simulink model "IEEE14_bus_system_2"  (R2024a)
settings: Solver=VariableStepAuto  StartTime=0.0  StopTime=0.2  RelTol=1e-3
libraries: spsThreePhaseSeriesRLCBranchLib x120, spsThreePhaseVIMeasurementLib x51, spsGroundLib x40, spsLoadFlowBusLib x33, spsThreePhaseSeriesRLCLoadLib x24, spsThreePhaseSourceLib x10, spsThreePhaseTransformerTwoWindingsLib x5, spspowerguiLib x2
(part 3 of 3)

== system IEEE14_bus_system_2/Line 4-3 ==
  B1 : spsThreePhaseSeriesRLCBranchLib/Three-Phase Series RLC Branch  LConnTagsString=A|B|C  RConnTagsString=A|B|C  BranchType=C  Resistance=1e-6  Inductance=1e-3  Capacitance=B/(2*pi*F)  Measurements=None
  B2 : spsThreePhaseSeriesRLCBranchLib/Three-Phase Series RLC Branch  LConnTagsString=A|B|C  RConnTagsString=A|B|C  BranchType=C  Resistance=1e-6  Inductance=1e-3  Capacitance=B/(2*pi*F)  Measurements=None
  Ground : spsGroundLib/Ground  LConnTagsString=a
  RL : spsThreePhaseSeriesRLCBranchLib/Three-Phase Series RLC Branch  LConnTagsString=A|B|C  RConnTagsString=A|B|C  BranchType=RL  Resistance=R  Inductance=xL/(2*pi*F)  Capacitance=1e-6  Measurements=None
  A : PMIOPort  Side=Left
  B : PMIOPort  Port=2  Side=Left
  C : PMIOPort  Port=3  Side=Left
  a : PMIOPort  Port=4  Side=Right
  b : PMIOPort  Port=5  Side=Right
  c : PMIOPort  Port=6  Side=Right
  connections:
  RL/LConn1 -- A/RConn1 -- B1/LConn1
  RL/RConn1 -- a/RConn1 -- B2/LConn1
  RL/LConn2 -- B/RConn1 -- B1/LConn2
  RL/RConn2 -- b/RConn1 -- B2/LConn2
  RL/RConn3 -- B2/LConn3 -- c/RConn1
  RL/LConn3 -- B1/LConn3 -- C/RConn1
  B1/RConn1 -- B1/RConn2 -- B1/RConn3 -- B2/RConn1 -- B2/RConn2 -- B2/RConn3 -- Ground/LConn1

== system IEEE14_bus_system_2/Line 4-5 ==
  B1 : spsThreePhaseSeriesRLCBranchLib/Three-Phase Series RLC Branch  LConnTagsString=A|B|C  RConnTagsString=A|B|C  BranchType=C  Resistance=0  Inductance=1e-3  Capacitance=B/(2*pi*F)  Measurements=None
  B2 : spsThreePhaseSeriesRLCBranchLib/Three-Phase Series RLC Branch  LConnTagsString=A|B|C  RConnTagsString=A|B|C  BranchType=C  Resistance=1e-6  Inductance=1e-3  Capacitance=B/(2*pi*F)  Measurements=None
  Ground : spsGroundLib/Ground  LConnTagsString=a
  RL : spsThreePhaseSeriesRLCBranchLib/Three-Phase Series RLC Branch  LConnTagsString=A|B|C  RConnTagsString=A|B|C  BranchType=RL  Resistance=R  Inductance=xL/(2*pi*F)  Capacitance=1e-6  Measurements=None
  A : PMIOPort  Side=Left
  B : PMIOPort  Port=2  Side=Left
  C : PMIOPort  Port=3  Side=Left
  a : PMIOPort  Port=4  Side=Right
  b : PMIOPort  Port=5  Side=Right
  c : PMIOPort  Port=6  Side=Right
  connections:
  RL/LConn1 -- A/RConn1 -- B1/LConn1
  RL/RConn1 -- a/RConn1 -- B2/LConn1
  RL/LConn2 -- B/RConn1 -- B1/LConn2
  RL/RConn2 -- b/RConn1 -- B2/LConn2
  RL/RConn3 -- B2/LConn3 -- c/RConn1
  RL/LConn3 -- B1/LConn3 -- C/RConn1
  B1/RConn1 -- B1/RConn2 -- B1/RConn3 -- B2/RConn1 -- B2/RConn2 -- B2/RConn3 -- Ground/LConn1

== system IEEE14_bus_system_2/Line 4-7 ==
  B1 : spsThreePhaseSeriesRLCBranchLib/Three-Phase Series RLC Branch  LConnTagsString=A|B|C  RConnTagsString=A|B|C  BranchType=C  Resistance=1e-6  Inductance=1e-3  Capacitance=B/(2*pi*F)  Measurements=None
  B2 : spsThreePhaseSeriesRLCBranchLib/Three-Phase Series RLC Branch  LConnTagsString=A|B|C  RConnTagsString=A|B|C  BranchType=C  Resistance=1e-6  Inductance=1e-3  Capacitance=B/(2*pi*F)  Measurements=None
  Ground : spsGroundLib/Ground  LConnTagsString=a
  RL : spsThreePhaseSeriesRLCBranchLib/Three-Phase Series RLC Branch  LConnTagsString=A|B|C  RConnTagsString=A|B|C  BranchType=RL  Resistance=R  Inductance=xL/(2*pi*F)  Capacitance=1e-6  Measurements=None
  A : PMIOPort  Side=Left
  B : PMIOPort  Port=2  Side=Left
  C : PMIOPort  Port=3  Side=Left
  a : PMIOPort  Port=4  Side=Right
  b : PMIOPort  Port=5  Side=Right
  c : PMIOPort  Port=6  Side=Right
  connections:
  RL/LConn1 -- A/RConn1 -- B1/LConn1
  RL/RConn1 -- a/RConn1 -- B2/LConn1
  RL/LConn2 -- B/RConn1 -- B1/LConn2
  RL/RConn2 -- b/RConn1 -- B2/LConn2
  RL/RConn3 -- B2/LConn3 -- c/RConn1
  RL/LConn3 -- B1/LConn3 -- C/RConn1
  B1/RConn1 -- B1/RConn2 -- B1/RConn3 -- B2/RConn1 -- B2/RConn2 -- B2/RConn3 -- Ground/LConn1

== system IEEE14_bus_system_2/Line 4-9 ==
  B1 : spsThreePhaseSeriesRLCBranchLib/Three-Phase Series RLC Branch  LConnTagsString=A|B|C  RConnTagsString=A|B|C  BranchType=C  Resistance=1e-6  Inductance=1e-3  Capacitance=B/(2*pi*F)  Measurements=None
  B2 : spsThreePhaseSeriesRLCBranchLib/Three-Phase Series RLC Branch  LConnTagsString=A|B|C  RConnTagsString=A|B|C  BranchType=C  Resistance=1e-6  Inductance=1e-3  Capacitance=B/(2*pi*F)  Measurements=None
  Ground : spsGroundLib/Ground  LConnTagsString=a
  RL : spsThreePhaseSeriesRLCBranchLib/Three-Phase Series RLC Branch  LConnTagsString=A|B|C  RConnTagsString=A|B|C  BranchType=RL  Resistance=R  Inductance=xL/(2*pi*F)  Capacitance=1e-6  Measurements=None
  A : PMIOPort  Side=Left
  B : PMIOPort  Port=2  Side=Left
  C : PMIOPort  Port=3  Side=Left
  a : PMIOPort  Port=4  Side=Right
  b : PMIOPort  Port=5  Side=Right
  c : PMIOPort  Port=6  Side=Right
  connections:
  RL/LConn1 -- A/RConn1 -- B1/LConn1
  RL/RConn1 -- a/RConn1 -- B2/LConn1
  RL/LConn2 -- B/RConn1 -- B1/LConn2
  RL/RConn2 -- b/RConn1 -- B2/LConn2
  RL/RConn3 -- B2/LConn3 -- c/RConn1
  RL/LConn3 -- B1/LConn3 -- C/RConn1
  B1/RConn1 -- B1/RConn2 -- B1/RConn3 -- B2/RConn1 -- B2/RConn2 -- B2/RConn3 -- Ground/LConn1

== system IEEE14_bus_system_2/Line 5-1 ==
  B1 : spsThreePhaseSeriesRLCBranchLib/Three-Phase Series RLC Branch  LConnTagsString=A|B|C  RConnTagsString=A|B|C  BranchType=C  Resistance=0  Inductance=1e-3  Capacitance=B/(2*pi*F)  Measurements=None
  B2 : spsThreePhaseSeriesRLCBranchLib/Three-Phase Series RLC Branch  LConnTagsString=A|B|C  RConnTagsString=A|B|C  BranchType=C  Resistance=1e-6  Inductance=1e-3  Capacitance=B/(2*pi*F)  Measurements=None
  Ground : spsGroundLib/Ground  LConnTagsString=a
  RL : spsThreePhaseSeriesRLCBranchLib/Three-Phase Series RLC Branch  LConnTagsString=A|B|C  RConnTagsString=A|B|C  BranchType=RL  Resistance=R  Inductance=xL/(2*pi*F)  Capacitance=1e-6  Measurements=None
  A : PMIOPort  Side=Left
  B : PMIOPort  Port=2  Side=Left
  C : PMIOPort  Port=3  Side=Left
  a : PMIOPort  Port=4  Side=Right
  b : PMIOPort  Port=5  Side=Right
  c : PMIOPort  Port=6  Side=Right
  connections:
  RL/LConn1 -- A/RConn1 -- B1/LConn1
  RL/RConn1 -- a/RConn1 -- B2/LConn1
  RL/LConn2 -- B/RConn1 -- B1/LConn2
  RL/RConn2 -- b/RConn1 -- B2/LConn2
  RL/RConn3 -- B2/LConn3 -- c/RConn1
  RL/LConn3 -- B1/LConn3 -- C/RConn1
  B1/RConn1 -- B1/RConn2 -- B1/RConn3 -- B2/RConn1 -- B2/RConn2 -- B2/RConn3 -- Ground/LConn1

== system IEEE14_bus_system_2/Line 5-6 ==
  B1 : spsThreePhaseSeriesRLCBranchLib/Three-Phase Series RLC Branch  LConnTagsString=A|B|C  RConnTagsString=A|B|C  BranchType=C  Resistance=0  Inductance=1e-3  Capacitance=B/(2*pi*F)  Measurements=None
  B2 : spsThreePhaseSeriesRLCBranchLib/Three-Phase Series RLC Branch  LConnTagsString=A|B|C  RConnTagsString=A|B|C  BranchType=C  Resistance=1e-6  Inductance=1e-3  Capacitance=B/(2*pi*F)  Measurements=None
  Ground : spsGroundLib/Ground  LConnTagsString=a
  RL : spsThreePhaseSeriesRLCBranchLib/Three-Phase Series RLC Branch  LConnTagsString=A|B|C  RConnTagsString=A|B|C  BranchType=RL  Resistance=R  Inductance=xL/(2*pi*F)  Capacitance=1e-6  Measurements=None
  A : PMIOPort  Side=Left
  B : PMIOPort  Port=2  Side=Left
  C : PMIOPort  Port=3  Side=Left
  a : PMIOPort  Port=4  Side=Right
  b : PMIOPort  Port=5  Side=Right
  c : PMIOPort  Port=6  Side=Right
  connections:
  RL/LConn1 -- A/RConn1 -- B1/LConn1
  RL/RConn1 -- a/RConn1 -- B2/LConn1
  RL/LConn2 -- B/RConn1 -- B1/LConn2
  RL/RConn2 -- b/RConn1 -- B2/LConn2
  RL/RConn3 -- B2/LConn3 -- c/RConn1
  RL/LConn3 -- B1/LConn3 -- C/RConn1
  B1/RConn1 -- B1/RConn2 -- B1/RConn3 -- B2/RConn1 -- B2/RConn2 -- B2/RConn3 -- Ground/LConn1

== system IEEE14_bus_system_2/Line 6-1 ==
  B1 : spsThreePhaseSeriesRLCBranchLib/Three-Phase Series RLC Branch  LConnTagsString=A|B|C  RConnTagsString=A|B|C  BranchType=C  Resistance=1e-6  Inductance=1e-3  Capacitance=B/(2*pi*F)  Measurements=None
  B2 : spsThreePhaseSeriesRLCBranchLib/Three-Phase Series RLC Branch  LConnTagsString=A|B|C  RConnTagsString=A|B|C  BranchType=C  Resistance=1e-6  Inductance=1e-3  Capacitance=B/(2*pi*F)  Measurements=None
  Ground : spsGroundLib/Ground  LConnTagsString=a
  RL : spsThreePhaseSeriesRLCBranchLib/Three-Phase Series RLC Branch  LConnTagsString=A|B|C  RConnTagsString=A|B|C  BranchType=RL  Resistance=R  Inductance=xL/(2*pi*F)  Capacitance=1e-6  Measurements=None
  A : PMIOPort  Side=Left
  B : PMIOPort  Port=2  Side=Left
  C : PMIOPort  Port=3  Side=Left
  a : PMIOPort  Port=4  Side=Right
  b : PMIOPort  Port=5  Side=Right
  c : PMIOPort  Port=6  Side=Right
  connections:
  RL/LConn1 -- A/RConn1 -- B1/LConn1
  RL/RConn1 -- a/RConn1 -- B2/LConn1
  RL/LConn2 -- B/RConn1 -- B1/LConn2
  RL/RConn2 -- b/RConn1 -- B2/LConn2
  RL/RConn3 -- B2/LConn3 -- c/RConn1
  RL/LConn3 -- B1/LConn3 -- C/RConn1
  B1/RConn1 -- B1/RConn2 -- B1/RConn3 -- B2/RConn1 -- B2/RConn2 -- B2/RConn3 -- Ground/LConn1

== system IEEE14_bus_system_2/Line 6-11 ==
  B1 : spsThreePhaseSeriesRLCBranchLib/Three-Phase Series RLC Branch  LConnTagsString=A|B|C  RConnTagsString=A|B|C  BranchType=C  Resistance=1e-6  Inductance=1e-3  Capacitance=B/(2*pi*F)  Measurements=None
  B2 : spsThreePhaseSeriesRLCBranchLib/Three-Phase Series RLC Branch  LConnTagsString=A|B|C  RConnTagsString=A|B|C  BranchType=C  Resistance=1e-6  Inductance=1e-3  Capacitance=B/(2*pi*F)  Measurements=None
  Ground : spsGroundLib/Ground  LConnTagsString=a
  RL : spsThreePhaseSeriesRLCBranchLib/Three-Phase Series RLC Branch  LConnTagsString=A|B|C  RConnTagsString=A|B|C  BranchType=RL  Resistance=R  Inductance=xL/(2*pi*F)  Capacitance=1e-6  Measurements=None
  A : PMIOPort  Side=Left
  B : PMIOPort  Port=2  Side=Left
  C : PMIOPort  Port=3  Side=Left
  a : PMIOPort  Port=4  Side=Right
  b : PMIOPort  Port=5  Side=Right
  c : PMIOPort  Port=6  Side=Right
  connections:
  RL/LConn1 -- A/RConn1 -- B1/LConn1
  RL/RConn1 -- a/RConn1 -- B2/LConn1
  RL/LConn2 -- B/RConn1 -- B1/LConn2
  RL/RConn2 -- b/RConn1 -- B2/LConn2
  RL/RConn3 -- B2/LConn3 -- c/RConn1
  RL/LConn3 -- B1/LConn3 -- C/RConn1
  B1/RConn1 -- B1/RConn2 -- B1/RConn3 -- B2/RConn1 -- B2/RConn2 -- B2/RConn3 -- Ground/LConn1

== system IEEE14_bus_system_2/Line 6-12 ==
  B1 : spsThreePhaseSeriesRLCBranchLib/Three-Phase Series RLC Branch  LConnTagsString=A|B|C  RConnTagsString=A|B|C  BranchType=C  Resistance=1e-6  Inductance=1e-3  Capacitance=B/(2*pi*F)  Measurements=None
  B2 : spsThreePhaseSeriesRLCBranchLib/Three-Phase Series RLC Branch  LConnTagsString=A|B|C  RConnTagsString=A|B|C  BranchType=C  Resistance=1e-6  Inductance=1e-3  Capacitance=B/(2*pi*F)  Measurements=None
  Ground : spsGroundLib/Ground  LConnTagsString=a
  RL : spsThreePhaseSeriesRLCBranchLib/Three-Phase Series RLC Branch  LConnTagsString=A|B|C  RConnTagsString=A|B|C  BranchType=RL  Resistance=R  Inductance=xL/(2*pi*F)  Capacitance=1e-6  Measurements=None
  A : PMIOPort  Side=Left
  B : PMIOPort  Port=2  Side=Left
  C : PMIOPort  Port=3  Side=Left
  a : PMIOPort  Port=4  Side=Right
  b : PMIOPort  Port=5  Side=Right
  c : PMIOPort  Port=6  Side=Right
  connections:
  RL/LConn1 -- A/RConn1 -- B1/LConn1
  RL/RConn1 -- a/RConn1 -- B2/LConn1
  RL/LConn2 -- B/RConn1 -- B1/LConn2
  RL/RConn2 -- b/RConn1 -- B2/LConn2
  RL/RConn3 -- B2/LConn3 -- c/RConn1
  RL/LConn3 -- B1/LConn3 -- C/RConn1
  B1/RConn1 -- B1/RConn2 -- B1/RConn3 -- B2/RConn1 -- B2/RConn2 -- B2/RConn3 -- Ground/LConn1

== system IEEE14_bus_system_2/Line 6-13 ==
  B1 : spsThreePhaseSeriesRLCBranchLib/Three-Phase Series RLC Branch  LConnTagsString=A|B|C  RConnTagsString=A|B|C  BranchType=C  Resistance=1e-6  Inductance=1e-3  Capacitance=B/(2*pi*F)  Measurements=None
  B2 : spsThreePhaseSeriesRLCBranchLib/Three-Phase Series RLC Branch  LConnTagsString=A|B|C  RConnTagsString=A|B|C  BranchType=C  Resistance=1e-6  Inductance=1e-3  Capacitance=B/(2*pi*F)  Measurements=None
  Ground : spsGroundLib/Ground  LConnTagsString=a
  RL : spsThreePhaseSeriesRLCBranchLib/Three-Phase Series RLC Branch  LConnTagsString=A|B|C  RConnTagsString=A|B|C  BranchType=RL  Resistance=R  Inductance=xL/(2*pi*F)  Capacitance=1e-6  Measurements=None
  A : PMIOPort  Side=Left
  B : PMIOPort  Port=2  Side=Left
  C : PMIOPort  Port=3  Side=Left
  a : PMIOPort  Port=4  Side=Right
  b : PMIOPort  Port=5  Side=Right
  c : PMIOPort  Port=6  Side=Right
  connections:
  RL/LConn1 -- A/RConn1 -- B1/LConn1
  RL/RConn1 -- a/RConn1 -- B2/LConn1
  RL/LConn2 -- B/RConn1 -- B1/LConn2
  RL/RConn2 -- b/RConn1 -- B2/LConn2
  RL/RConn3 -- B2/LConn3 -- c/RConn1
  RL/LConn3 -- B1/LConn3 -- C/RConn1
  B1/RConn1 -- B1/RConn2 -- B1/RConn3 -- B2/RConn1 -- B2/RConn2 -- B2/RConn3 -- Ground/LConn1

== system IEEE14_bus_system_2/Line 6-2 ==
  B1 : spsThreePhaseSeriesRLCBranchLib/Three-Phase Series RLC Branch  LConnTagsString=A|B|C  RConnTagsString=A|B|C  BranchType=C  Resistance=1e-6  Inductance=1e-3  Capacitance=B/(2*pi*F)  Measurements=None
  B2 : spsThreePhaseSeriesRLCBranchLib/Three-Phase Series RLC Branch  LConnTagsString=A|B|C  RConnTagsString=A|B|C  BranchType=C  Resistance=1e-6  Inductance=1e-3  Capacitance=B/(2*pi*F)  Measurements=None
  Ground : spsGroundLib/Ground  LConnTagsString=a
  RL : spsThreePhaseSeriesRLCBranchLib/Three-Phase Series RLC Branch  LConnTagsString=A|B|C  RConnTagsString=A|B|C  BranchType=RL  Resistance=R  Inductance=xL/(2*pi*F)  Capacitance=1e-6  Measurements=None
  A : PMIOPort  Side=Left
  B : PMIOPort  Port=2  Side=Left
  C : PMIOPort  Port=3  Side=Left
  a : PMIOPort  Port=4  Side=Right
  b : PMIOPort  Port=5  Side=Right
  c : PMIOPort  Port=6  Side=Right
  connections:
  RL/LConn1 -- A/RConn1 -- B1/LConn1
  RL/RConn1 -- a/RConn1 -- B2/LConn1
  RL/LConn2 -- B/RConn1 -- B1/LConn2
  RL/RConn2 -- b/RConn1 -- B2/LConn2
  RL/RConn3 -- B2/LConn3 -- c/RConn1
  RL/LConn3 -- B1/LConn3 -- C/RConn1
  B1/RConn1 -- B1/RConn2 -- B1/RConn3 -- B2/RConn1 -- B2/RConn2 -- B2/RConn3 -- Ground/LConn1

== system IEEE14_bus_system_2/Line 6-3 ==
  B1 : spsThreePhaseSeriesRLCBranchLib/Three-Phase Series RLC Branch  LConnTagsString=A|B|C  RConnTagsString=A|B|C  BranchType=C  Resistance=1e-6  Inductance=1e-3  Capacitance=B/(2*pi*F)  Measurements=None
  B2 : spsThreePhaseSeriesRLCBranchLib/Three-Phase Series RLC Branch  LConnTagsString=A|B|C  RConnTagsString=A|B|C  BranchType=C  Resistance=1e-6  Inductance=1e-3  Capacitance=B/(2*pi*F)  Measurements=None
  Ground : spsGroundLib/Ground  LConnTagsString=a
  RL : spsThreePhaseSeriesRLCBranchLib/Three-Phase Series RLC Branch  LConnTagsString=A|B|C  RConnTagsString=A|B|C  BranchType=RL  Resistance=R  Inductance=xL/(2*pi*F)  Capacitance=1e-6  Measurements=None
  A : PMIOPort  Side=Left
  B : PMIOPort  Port=2  Side=Left
  C : PMIOPort  Port=3  Side=Left
  a : PMIOPort  Port=4  Side=Right
  b : PMIOPort  Port=5  Side=Right
  c : PMIOPort  Port=6  Side=Right
  connections:
  RL/LConn1 -- A/RConn1 -- B1/LConn1
  RL/RConn1 -- a/RConn1 -- B2/LConn1
  RL/LConn2 -- B/RConn1 -- B1/LConn2
  RL/RConn2 -- b/RConn1 -- B2/LConn2
  RL/RConn3 -- B2/LConn3 -- c/RConn1
  RL/LConn3 -- B1/LConn3 -- C/RConn1
  B1/RConn1 -- B1/RConn2 -- B1/RConn3 -- B2/RConn1 -- B2/RConn2 -- B2/RConn3 -- Ground/LConn1

== system IEEE14_bus_system_2/Line 7-1 ==
  B1 : spsThreePhaseSeriesRLCBranchLib/Three-Phase Series RLC Branch  LConnTagsString=A|B|C  RConnTagsString=A|B|C  BranchType=C  Resistance=1e-6  Inductance=1e-3  Capacitance=B/(2*pi*F)  Measurements=None
  B2 : spsThreePhaseSeriesRLCBranchLib/Three-Phase Series RLC Branch  LConnTagsString=A|B|C  RConnTagsString=A|B|C  BranchType=C  Resistance=1e-6  Inductance=1e-3  Capacitance=B/(2*pi*F)  Measurements=None
  Ground : spsGroundLib/Ground  LConnTagsString=a
  RL : spsThreePhaseSeriesRLCBranchLib/Three-Phase Series RLC Branch  LConnTagsString=A|B|C  RConnTagsString=A|B|C  BranchType=RL  Resistance=R  Inductance=xL/(2*pi*F)  Capacitance=1e-6  Measurements=None
  A : PMIOPort  Side=Left
  B : PMIOPort  Port=2  Side=Left
  C : PMIOPort  Port=3  Side=Left
  a : PMIOPort  Port=4  Side=Right
  b : PMIOPort  Port=5  Side=Right
  c : PMIOPort  Port=6  Side=Right
  connections:
  RL/LConn1 -- A/RConn1 -- B1/LConn1
  RL/RConn1 -- a/RConn1 -- B2/LConn1
  RL/LConn2 -- B/RConn1 -- B1/LConn2
  RL/RConn2 -- b/RConn1 -- B2/LConn2
  RL/RConn3 -- B2/LConn3 -- c/RConn1
  RL/LConn3 -- B1/LConn3 -- C/RConn1
  B1/RConn1 -- B1/RConn2 -- B1/RConn3 -- B2/RConn1 -- B2/RConn2 -- B2/RConn3 -- Ground/LConn1

== system IEEE14_bus_system_2/Line 7-2 ==
  B1 : spsThreePhaseSeriesRLCBranchLib/Three-Phase Series RLC Branch  LConnTagsString=A|B|C  RConnTagsString=A|B|C  BranchType=C  Resistance=1e-6  Inductance=1e-3  Capacitance=B/(2*pi*F)  Measurements=None
  B2 : spsThreePhaseSeriesRLCBranchLib/Three-Phase Series RLC Branch  LConnTagsString=A|B|C  RConnTagsString=A|B|C  BranchType=C  Resistance=1e-6  Inductance=1e-3  Capacitance=B/(2*pi*F)  Measurements=None
  Ground : spsGroundLib/Ground  LConnTagsString=a
  RL : spsThreePhaseSeriesRLCBranchLib/Three-Phase Series RLC Branch  LConnTagsString=A|B|C  RConnTagsString=A|B|C  BranchType=RL  Resistance=R  Inductance=xL/(2*pi*F)  Capacitance=1e-6  Measurements=None
  A : PMIOPort  Side=Left
  B : PMIOPort  Port=2  Side=Left
  C : PMIOPort  Port=3  Side=Left
  a : PMIOPort  Port=4  Side=Right
  b : PMIOPort  Port=5  Side=Right
  c : PMIOPort  Port=6  Side=Right
  connections:
  RL/LConn1 -- A/RConn1 -- B1/LConn1
  RL/RConn1 -- a/RConn1 -- B2/LConn1
  RL/LConn2 -- B/RConn1 -- B1/LConn2
  RL/RConn2 -- b/RConn1 -- B2/LConn2
  RL/RConn3 -- B2/LConn3 -- c/RConn1
  RL/LConn3 -- B1/LConn3 -- C/RConn1
  B1/RConn1 -- B1/RConn2 -- B1/RConn3 -- B2/RConn1 -- B2/RConn2 -- B2/RConn3 -- Ground/LConn1

== system IEEE14_bus_system_2/Line 7-8 ==
  B1 : spsThreePhaseSeriesRLCBranchLib/Three-Phase Series RLC Branch  LConnTagsString=A|B|C  RConnTagsString=A|B|C  BranchType=C  Resistance=1e-6  Inductance=1e-3  Capacitance=B/(2*pi*F)  Measurements=None
  B2 : spsThreePhaseSeriesRLCBranchLib/Three-Phase Series RLC Branch  LConnTagsString=A|B|C  RConnTagsString=A|B|C  BranchType=C  Resistance=1e-6  Inductance=1e-3  Capacitance=B/(2*pi*F)  Measurements=None
  Ground : spsGroundLib/Ground  LConnTagsString=a
  RL : spsThreePhaseSeriesRLCBranchLib/Three-Phase Series RLC Branch  LConnTagsString=A|B|C  RConnTagsString=A|B|C  BranchType=RL  Resistance=R  Inductance=xL/(2*pi*F)  Capacitance=1e-6  Measurements=None
  A : PMIOPort  Side=Left
  B : PMIOPort  Port=2  Side=Left
  C : PMIOPort  Port=3  Side=Left
  a : PMIOPort  Port=4  Side=Right
  b : PMIOPort  Port=5  Side=Right
  c : PMIOPort  Port=6  Side=Right
  connections:
  RL/LConn1 -- A/RConn1 -- B1/LConn1
  RL/RConn1 -- a/RConn1 -- B2/LConn1
  RL/LConn2 -- B/RConn1 -- B1/LConn2
  RL/RConn2 -- b/RConn1 -- B2/LConn2
  RL/RConn3 -- B2/LConn3 -- c/RConn1
  RL/LConn3 -- B1/LConn3 -- C/RConn1
  B1/RConn1 -- B1/RConn2 -- B1/RConn3 -- B2/RConn1 -- B2/RConn2 -- B2/RConn3 -- Ground/LConn1

== system IEEE14_bus_system_2/Line 7-9 ==
  B1 : spsThreePhaseSeriesRLCBranchLib/Three-Phase Series RLC Branch  LConnTagsString=A|B|C  RConnTagsString=A|B|C  BranchType=C  Resistance=1e-6  Inductance=1e-3  Capacitance=B/(2*pi*F)  Measurements=None
  B2 : spsThreePhaseSeriesRLCBranchLib/Three-Phase Series RLC Branch  LConnTagsString=A|B|C  RConnTagsString=A|B|C  BranchType=C  Resistance=1e-6  Inductance=1e-3  Capacitance=B/(2*pi*F)  Measurements=None
  Ground : spsGroundLib/Ground  LConnTagsString=a
  RL : spsThreePhaseSeriesRLCBranchLib/Three-Phase Series RLC Branch  LConnTagsString=A|B|C  RConnTagsString=A|B|C  BranchType=RL  Resistance=R  Inductance=xL/(2*pi*F)  Capacitance=1e-6  Measurements=None
  A : PMIOPort  Side=Left
  B : PMIOPort  Port=2  Side=Left
  C : PMIOPort  Port=3  Side=Left
  a : PMIOPort  Port=4  Side=Right
  b : PMIOPort  Port=5  Side=Right
  c : PMIOPort  Port=6  Side=Right
  connections:
  RL/LConn1 -- A/RConn1 -- B1/LConn1
  RL/RConn1 -- a/RConn1 -- B2/LConn1
  RL/LConn2 -- B/RConn1 -- B1/LConn2
  RL/RConn2 -- b/RConn1 -- B2/LConn2
  RL/RConn3 -- B2/LConn3 -- c/RConn1
  RL/LConn3 -- B1/LConn3 -- C/RConn1
  B1/RConn1 -- B1/RConn2 -- B1/RConn3 -- B2/RConn1 -- B2/RConn2 -- B2/RConn3 -- Ground/LConn1

== system IEEE14_bus_system_2/Line 9-1 ==
  B1 : spsThreePhaseSeriesRLCBranchLib/Three-Phase Series RLC Branch  LConnTagsString=A|B|C  RConnTagsString=A|B|C  BranchType=C  Resistance=1e-6  Inductance=1e-3  Capacitance=B/(2*pi*F)  Measurements=None
  B2 : spsThreePhaseSeriesRLCBranchLib/Three-Phase Series RLC Branch  LConnTagsString=A|B|C  RConnTagsString=A|B|C  BranchType=C  Resistance=1e-6  Inductance=1e-3  Capacitance=B/(2*pi*F)  Measurements=None
  Ground : spsGroundLib/Ground  LConnTagsString=a
  RL : spsThreePhaseSeriesRLCBranchLib/Three-Phase Series RLC Branch  LConnTagsString=A|B|C  RConnTagsString=A|B|C  BranchType=RL  Resistance=R  Inductance=xL/(2*pi*F)  Capacitance=1e-6  Measurements=None
  A : PMIOPort  Side=Left
  B : PMIOPort  Port=2  Side=Left
  C : PMIOPort  Port=3  Side=Left
  a : PMIOPort  Port=4  Side=Right
  b : PMIOPort  Port=5  Side=Right
  c : PMIOPort  Port=6  Side=Right
  connections:
  RL/LConn1 -- A/RConn1 -- B1/LConn1
  RL/RConn1 -- a/RConn1 -- B2/LConn1
  RL/LConn2 -- B/RConn1 -- B1/LConn2
  RL/RConn2 -- b/RConn1 -- B2/LConn2
  RL/RConn3 -- B2/LConn3 -- c/RConn1
  RL/LConn3 -- B1/LConn3 -- C/RConn1
  B1/RConn1 -- B1/RConn2 -- B1/RConn3 -- B2/RConn1 -- B2/RConn2 -- B2/RConn3 -- Ground/LConn1

== system IEEE14_bus_system_2/Line 9-10 ==
  B1 : spsThreePhaseSeriesRLCBranchLib/Three-Phase Series RLC Branch  LConnTagsString=A|B|C  RConnTagsString=A|B|C  BranchType=C  Resistance=1e-6  Inductance=1e-3  Capacitance=B/(2*pi*F)  Measurements=None
  B2 : spsThreePhaseSeriesRLCBranchLib/Three-Phase Series RLC Branch  LConnTagsString=A|B|C  RConnTagsString=A|B|C  BranchType=C  Resistance=1e-6  Inductance=1e-3  Capacitance=B/(2*pi*F)  Measurements=None
  Ground : spsGroundLib/Ground  LConnTagsString=a
  RL : spsThreePhaseSeriesRLCBranchLib/Three-Phase Series RLC Branch  LConnTagsString=A|B|C  RConnTagsString=A|B|C  BranchType=RL  Resistance=R  Inductance=xL/(2*pi*F)  Capacitance=1e-6  Measurements=None
  A : PMIOPort  Side=Left
  B : PMIOPort  Port=2  Side=Left
  C : PMIOPort  Port=3  Side=Left
  a : PMIOPort  Port=4  Side=Right
  b : PMIOPort  Port=5  Side=Right
  c : PMIOPort  Port=6  Side=Right
  connections:
  RL/LConn1 -- A/RConn1 -- B1/LConn1
  RL/RConn1 -- a/RConn1 -- B2/LConn1
  RL/LConn2 -- B/RConn1 -- B1/LConn2
  RL/RConn2 -- b/RConn1 -- B2/LConn2
  RL/RConn3 -- B2/LConn3 -- c/RConn1
  RL/LConn3 -- B1/LConn3 -- C/RConn1
  B1/RConn1 -- B1/RConn2 -- B1/RConn3 -- B2/RConn1 -- B2/RConn2 -- B2/RConn3 -- Ground/LConn1

== system IEEE14_bus_system_2/Line 9-14 ==
  B1 : spsThreePhaseSeriesRLCBranchLib/Three-Phase Series RLC Branch  LConnTagsString=A|B|C  RConnTagsString=A|B|C  BranchType=C  Resistance=1e-6  Inductance=1e-3  Capacitance=B/(2*pi*F)  Measurements=None
  B2 : spsThreePhaseSeriesRLCBranchLib/Three-Phase Series RLC Branch  LConnTagsString=A|B|C  RConnTagsString=A|B|C  BranchType=C  Resistance=1e-6  Inductance=1e-3  Capacitance=B/(2*pi*F)  Measurements=None
  Ground : spsGroundLib/Ground  LConnTagsString=a
  RL : spsThreePhaseSeriesRLCBranchLib/Three-Phase Series RLC Branch  LConnTagsString=A|B|C  RConnTagsString=A|B|C  BranchType=RL  Resistance=R  Inductance=xL/(2*pi*F)  Capacitance=1e-6  Measurements=None
  A : PMIOPort  Side=Left
  B : PMIOPort  Port=2  Side=Left
  C : PMIOPort  Port=3  Side=Left
  a : PMIOPort  Port=4  Side=Right
  b : PMIOPort  Port=5  Side=Right
  c : PMIOPort  Port=6  Side=Right
  connections:
  RL/LConn1 -- A/RConn1 -- B1/LConn1
  RL/RConn1 -- a/RConn1 -- B2/LConn1
  RL/LConn2 -- B/RConn1 -- B1/LConn2
  RL/RConn2 -- b/RConn1 -- B2/LConn2
  RL/RConn3 -- B2/LConn3 -- c/RConn1
  RL/LConn3 -- B1/LConn3 -- C/RConn1
  B1/RConn1 -- B1/RConn2 -- B1/RConn3 -- B2/RConn1 -- B2/RConn2 -- B2/RConn3 -- Ground/LConn1

== system IEEE14_bus_system_2/Line 9-2 ==
  B1 : spsThreePhaseSeriesRLCBranchLib/Three-Phase Series RLC Branch  LConnTagsString=A|B|C  RConnTagsString=A|B|C  BranchType=C  Resistance=1e-6  Inductance=1e-3  Capacitance=B/(2*pi*F)  Measurements=None
  B2 : spsThreePhaseSeriesRLCBranchLib/Three-Phase Series RLC Branch  LConnTagsString=A|B|C  RConnTagsString=A|B|C  BranchType=C  Resistance=1e-6  Inductance=1e-3  Capacitance=B/(2*pi*F)  Measurements=None
  Ground : spsGroundLib/Ground  LConnTagsString=a
  RL : spsThreePhaseSeriesRLCBranchLib/Three-Phase Series RLC Branch  LConnTagsString=A|B|C  RConnTagsString=A|B|C  BranchType=RL  Resistance=R  Inductance=xL/(2*pi*F)  Capacitance=1e-6  Measurements=None
  A : PMIOPort  Side=Left
  B : PMIOPort  Port=2  Side=Left
  C : PMIOPort  Port=3  Side=Left
  a : PMIOPort  Port=4  Side=Right
  b : PMIOPort  Port=5  Side=Right
  c : PMIOPort  Port=6  Side=Right
  connections:
  RL/LConn1 -- A/RConn1 -- B1/LConn1
  RL/RConn1 -- a/RConn1 -- B2/LConn1
  RL/LConn2 -- B/RConn1 -- B1/LConn2
  RL/RConn2 -- b/RConn1 -- B2/LConn2
  RL/RConn3 -- B2/LConn3 -- c/RConn1
  RL/LConn3 -- B1/LConn3 -- C/RConn1
  B1/RConn1 -- B1/RConn2 -- B1/RConn3 -- B2/RConn1 -- B2/RConn2 -- B2/RConn3 -- Ground/LConn1
